simulink model "PMSM_MaxEfficiency"  (R2015a)
settings: Solver=ode45  StartTime=0.0  StopTime=5  RelTol=1e-3
values from neighbouring files (symbols this model uses):
  Ld = 0.00019    [aaa.mat]    (also in param.m = 2e-05)
  Lq = 0.00051    [aaa.mat]    (also in param.m = 4e-05)
  Pn = 4    [param.m]
  R = 2e-3    (= 0.002)    [param.m]
undefined symbols (not defined in the file or in its folder): D, Ia_vec, J, Phia, torque_vec
settings Model: Creator=hamada  LastModifiedBy=hamada

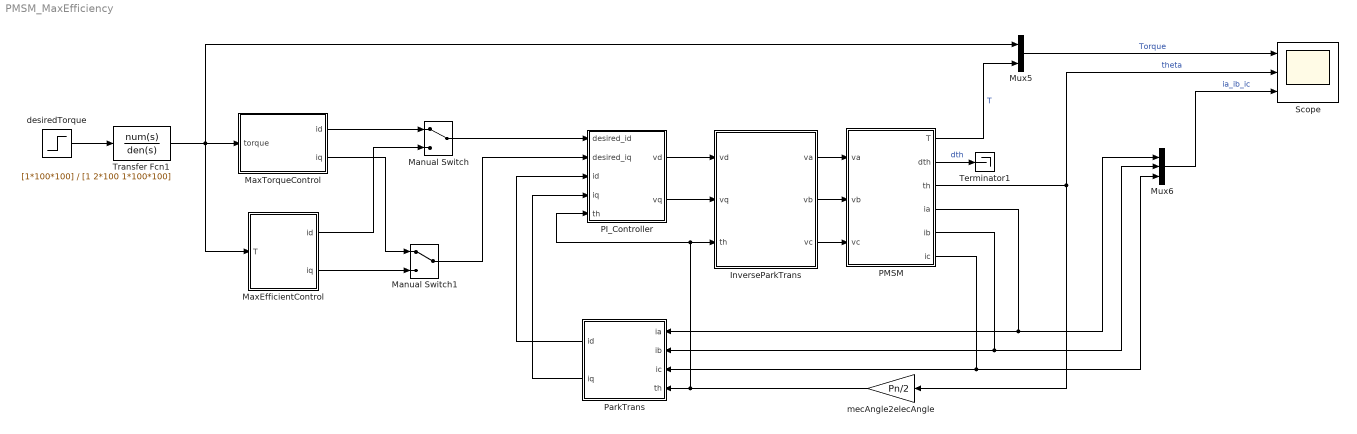
== system PMSM_MaxEfficiency ==
  InverseParkTrans : MATLAB Function  TreatAsAtomicUnit=on  SystemSampleTime=0.001
  Manual Switch : ManualSwitch
  Manual Switch1 : ManualSwitch
  MaxEfficientControl : MATLAB Function  TreatAsAtomicUnit=on  SystemSampleTime=0.001
  MaxTorqueControl : Subsystem
  Mux5 : Mux  Inputs=2
  Mux6 : Mux  Inputs=3
  PI_Controller : Subsystem  SystemSampleTime=0.001
  PMSM : Subsystem
  ParkTrans : MATLAB Function  TreatAsAtomicUnit=on
  Scope : Scope  NumInputPorts=3
      settings: TimeRange=5  YMin=0~0~-80  YMax=5~15~80
  Terminator1 : Terminator
  Transfer Fcn1 : TransferFcn  Numerator=[1*100*100]  Denominator=[1 2*100 1*100*100]
  desiredTorque : Step  After=5  SampleTime=0
  mecAngle2elecAngle : Gain  Gain=Pn/2
  wires:
  desiredTorque/1 -> Transfer Fcn1/1
  PMSM/1(T) -> Mux5/2  "T"
  PMSM/3(th) -> mecAngle2elecAngle/1, Scope/2  "theta"
  PMSM/4(ia) -> Mux6/1, ParkTrans/1(ia)
  PMSM/5(ib) -> ParkTrans/2(ib), Mux6/2
  PMSM/6(ic) -> ParkTrans/3(ic), Mux6/3
  InverseParkTrans/2(vb) -> PMSM/2(vb)
  InverseParkTrans/3(vc) -> PMSM/3(vc)
  InverseParkTrans/1(va) -> PMSM/1(va)
  mecAngle2elecAngle/1 -> ParkTrans/4(th), PI_Controller/5(th), InverseParkTrans/3(th)
  ParkTrans/1(id) -> PI_Controller/3(id)
  ParkTrans/2(iq) -> PI_Controller/4(iq)
  PI_Controller/1(vd) -> InverseParkTrans/1(vd)
  PI_Controller/2(vq) -> InverseParkTrans/2(vq)
  PMSM/2(dth) -> Terminator1/1  "dth"
  Mux5/1 -> Scope/1  "Torque"
  Mux6/1 -> Scope/3  "ia_ib_ic"
  Transfer Fcn1/1 -> MaxEfficientControl/1(T), MaxTorqueControl/1(torque), Mux5/1
  Manual Switch/1 -> PI_Controller/1(desired_id)
  MaxEfficientControl/2(iq) -> Manual Switch1/2
  MaxEfficientControl/1(id) -> Manual Switch/2
  MaxTorqueControl/1(id) -> Manual Switch/1
  MaxTorqueControl/2(iq) -> Manual Switch1/1
  Manual Switch1/1 -> PI_Controller/2(desired_iq)

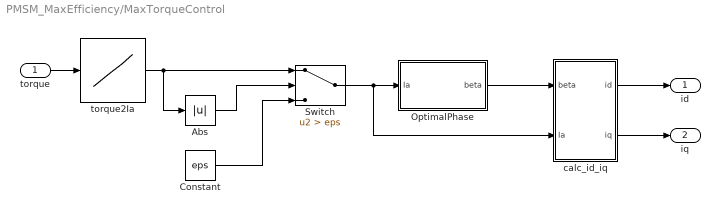
== system PMSM_MaxEfficiency/MaxTorqueControl ==
  torque : Inport
  Abs : Abs
  Constant : Constant  Value=eps
  OptimalPhase : Subsystem
  Switch : Switch  Criteria=u2 > Threshold  Threshold=eps
  calc_id_iq : Subsystem
  torque2Ia : Lookup_n-D  NumberOfTableDimensions=1  BreakpointsForDimension1=torque_vec  Table=Ia_vec  InternalRulePriority=Speed  RndMeth=Simplest  InputSameDT=on
  id : Outport
  iq : Outport  Port=2
  wires:
  torque/1 -> torque2Ia/1
  OptimalPhase/1(beta) -> calc_id_iq/1(beta)
  calc_id_iq/1(id) -> id/1
  calc_id_iq/2(iq) -> iq/1
  torque2Ia/1 -> Switch/1, Abs/1
  Abs/1 -> Switch/2
  Switch/1 -> calc_id_iq/2(Ia), OptimalPhase/1(Ia)
  Constant/1 -> Switch/3

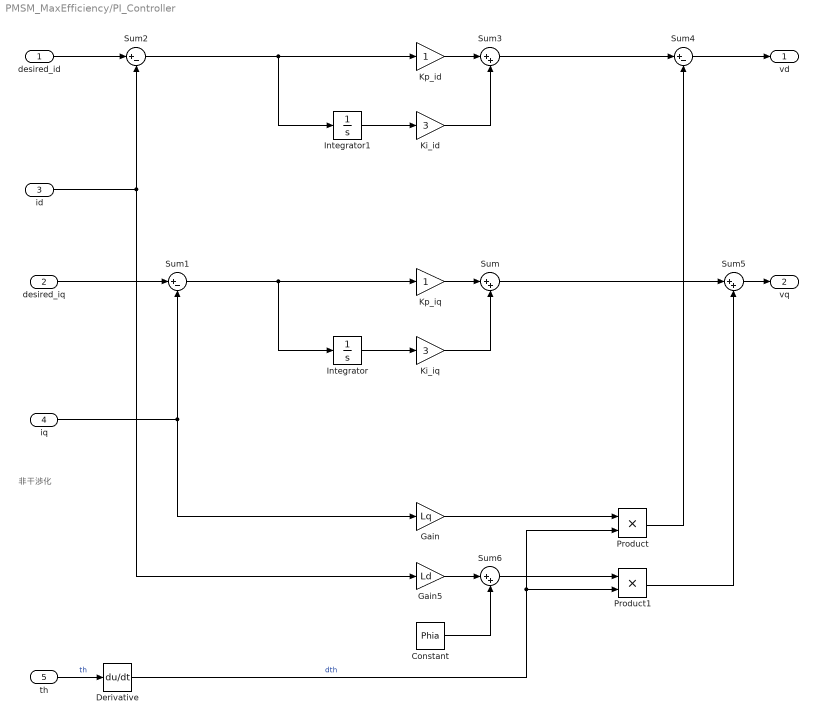
== system PMSM_MaxEfficiency/PI_Controller ==
  note: 非干渉化
  desired_id : Inport
  desired_iq : Inport  Port=2
  id : Inport  Port=3
  iq : Inport  Port=4
  th : Inport  Port=5
  Constant : Constant  Value=Phia
  Derivative : Derivative
  Gain : Gain  Gain=Lq
  Gain5 : Gain  Gain=Ld
  Integrator : Integrator
  Integrator1 : Integrator
  Ki_id : Gain  Gain=3
  Ki_iq : Gain  Gain=3
  Kp_id : Gain
  Kp_iq : Gain
  Product : Product
  Product1 : Product
  Sum{,3,5..6} (4 alike) : Sum  Inputs=|++
  Sum1 : Sum  Inputs=|+-
  Sum2 : Sum  Inputs=|+-
  Sum4 : Sum  Inputs=|+-
  vd : Outport
  vq : Outport  Port=2
  wires:
  Sum1/1 -> Integrator/1, Kp_iq/1
  desired_id/1 -> Sum2/1
  Kp_iq/1 -> Sum/1
  desired_iq/1 -> Sum1/1
  id/1 -> Sum2/2, Gain5/1
  iq/1 -> Sum1/2, Gain/1
  Sum/1 -> Sum5/1
  Integrator/1 -> Ki_iq/1
  Ki_iq/1 -> Sum/2
  Sum2/1 -> Integrator1/1, Kp_id/1
  Kp_id/1 -> Sum3/1
  Sum3/1 -> Sum4/1
  Integrator1/1 -> Ki_id/1
  Ki_id/1 -> Sum3/2
  th/1 -> Derivative/1  "th"
  Derivative/1 -> Product/2, Product1/2  "dth"
  Gain/1 -> Product/1
  Product/1 -> Sum4/2
  Sum4/1 -> vd/1
  Sum5/1 -> vq/1
  Gain5/1 -> Sum6/1
  Constant/1 -> Sum6/2
  Sum6/1 -> Product1/1
  Product1/1 -> Sum5/2

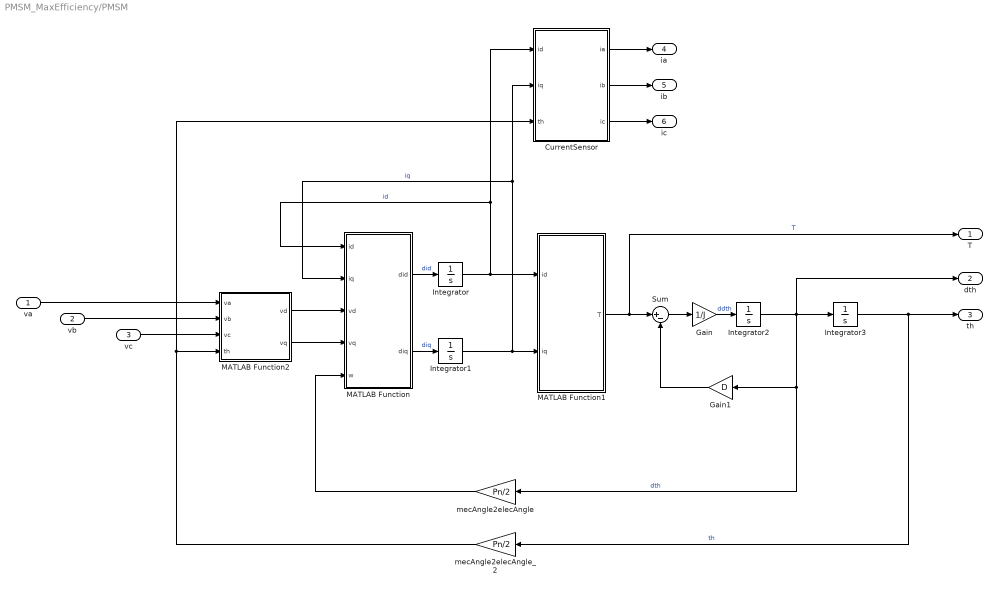
== system PMSM_MaxEfficiency/PMSM ==
  va : Inport
  vb : Inport  Port=2
  vc : Inport  Port=3
  CurrentSensor : MATLAB Function  TreatAsAtomicUnit=on
  Gain : Gain  Gain=1/J
  Gain1 : Gain  Gain=D
  Integrator{,1..3} (4 alike) : Integrator
  MATLAB Function : MATLAB Function  TreatAsAtomicUnit=on
  MATLAB Function1 : MATLAB Function  TreatAsAtomicUnit=on
  MATLAB Function2 : MATLAB Function  TreatAsAtomicUnit=on
  Sum : Sum  Inputs=|+-
  mecAngle2elecAngle : Gain  Gain=Pn/2
  mecAngle2elecAngle_2 : Gain  Gain=Pn/2
  T : Outport
  dth : Outport  Port=2
  th : Outport  Port=3
  ia : Outport  Port=4
  ib : Outport  Port=5
  ic : Outport  Port=6
  wires:
  CurrentSensor/3(ic) -> ic/1
  CurrentSensor/2(ib) -> ib/1
  CurrentSensor/1(ia) -> ia/1
  mecAngle2elecAngle_2/1 -> MATLAB Function2/4(th), CurrentSensor/3(th)
  mecAngle2elecAngle/1 -> MATLAB Function/5(w)
  Integrator3/1 -> mecAngle2elecAngle_2/1, th/1  "th"
  MATLAB Function2/2(vq) -> MATLAB Function/4(vq)
  MATLAB Function2/1(vd) -> MATLAB Function/3(vd)
  Gain1/1 -> Sum/2
  Integrator2/1 -> Gain1/1, mecAngle2elecAngle/1, Integrator3/1, dth/1  "dth"
  MATLAB Function1/1(T) -> Sum/1, T/1  "T"
  Gain/1 -> Integrator2/1  "ddth"
  Sum/1 -> Gain/1
  Integrator1/1 -> MATLAB Function1/2(iq), MATLAB Function/2(iq), CurrentSensor/2(iq)  "iq"
  Integrator/1 -> MATLAB Function1/1(id), MATLAB Function/1(id), CurrentSensor/1(id)  "id"
  MATLAB Function/2(diq) -> Integrator1/1  "diq"
  MATLAB Function/1(did) -> Integrator/1  "did"
  vc/1 -> MATLAB Function2/3(vc)
  vb/1 -> MATLAB Function2/2(vb)
  va/1 -> MATLAB Function2/1(va)

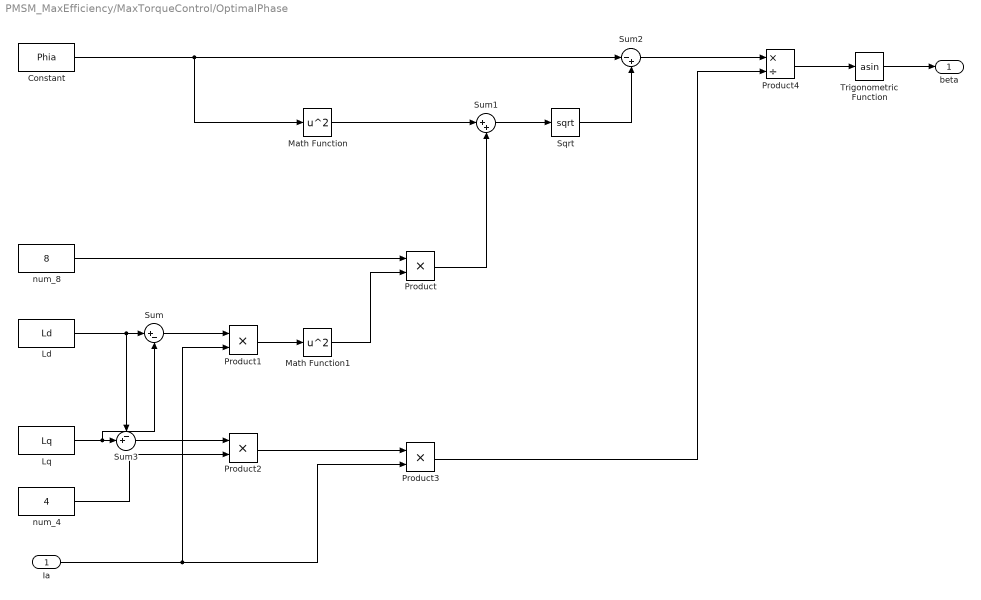
== system PMSM_MaxEfficiency/MaxTorqueControl/OptimalPhase ==
  Ia : Inport
  Constant : Constant  Value=Phia
  Ld : Constant  Value=Ld
  Lq : Constant  Value=Lq
  Math Function : Math  Operator=square  SaturateOnIntegerOverflow=on
  Math Function1 : Math  Operator=square  SaturateOnIntegerOverflow=on
  Product{,1..3} (4 alike) : Product
  Product4 : Product  Inputs=*/
  Sqrt : Sqrt  SaturateOnIntegerOverflow=on
  Sum : Sum  Inputs=|+-
  Sum1 : Sum  Inputs=|++
  Sum2 : Sum  Inputs=|-+
  Sum3 : Sum  Inputs=-+|
  Trigonometric Function : Trigonometry  Operator=asin
  num_4 : Constant  Value=4
  num_8 : Constant  Value=8
  beta : Outport
  wires:
  Constant/1 -> Sum2/1, Math Function/1
  Ld/1 -> Sum/1, Sum3/1
  Lq/1 -> Sum/2, Sum3/2
  Sum/1 -> Product1/1
  num_8/1 -> Product/1
  Math Function1/1 -> Product/2
  Product1/1 -> Math Function1/1
  Math Function/1 -> Sum1/1
  Product/1 -> Sum1/2
  Sum1/1 -> Sqrt/1
  Sqrt/1 -> Sum2/2
  Sum2/1 -> Product4/1
  Sum3/1 -> Product2/1
  Product2/1 -> Product3/1
  Ia/1 -> Product1/2, Product3/2
  num_4/1 -> Product2/2
  Product3/1 -> Product4/2
  Product4/1 -> Trigonometric Function/1
  Trigonometric Function/1 -> beta/1

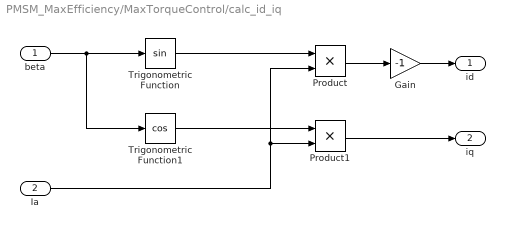
== system PMSM_MaxEfficiency/MaxTorqueControl/calc_id_iq ==
  beta : Inport
  Ia : Inport  Port=2
  Gain : Gain  Gain=-1
  Product : Product
  Product1 : Product
  Trigonometric Function : Trigonometry
  Trigonometric Function1 : Trigonometry  Operator=cos
  id : Outport
  iq : Outport  Port=2
  wires:
  Product/1 -> Gain/1
  beta/1 -> Trigonometric Function1/1, Trigonometric Function/1
  Trigonometric Function/1 -> Product/1
  Ia/1 -> Product1/2, Product/2
  Trigonometric Function1/1 -> Product1/1
  Product1/1 -> iq/1
  Gain/1 -> id/1

== matlab function PMSM_MaxEfficiency/InverseParkTrans ==
  data: vd input; vq input; va output; vb output; vc output; th input
function [ va, vb, vc ] = fcn( vd, vq, th ) 
    %#codegen
    buff = [
        cos( th ), -sin( th ), ( 1 / sqrt( 2 ) );
        cos( th - ( ( 2 * pi ) / 3 ) ), -sin( th - ( ( 2 * pi ) / 3 ) ), ( 1 / sqrt( 2 ) );
        cos( th + ( ( 2 * pi ) / 3 ) ), -sin( th + ( ( 2 * pi ) / 3 ) ), ( 1 / sqrt( 2 ) );
    ];

    vabc = sqrt( 2 / 3 ) * buff * [ vd;vq;0; ];
    va = vabc(1);
    vb = vabc(2);
    vc = vabc(3);
end

== matlab function PMSM_MaxEfficiency/ParkTrans ==
  data: ia input; ib input; ic input; th input; id output; iq output
function [ id, iq ] = fcn( ia, ib, ic, th ) 
    %#codegen
    buff = [
         cos( th ),  cos( th - ( ( 2 * pi ) / 3 ) ),  cos( th + ( ( 2 * pi ) / 3 ) );
        -sin( th ), -sin( th - ( ( 2 * pi ) / 3 ) ), -sin( th + ( ( 2 * pi ) / 3 ) );
        ( 1 / sqrt( 2 ) ), ( 1 / sqrt( 2 ) ), ( 1 / sqrt( 2 ) );
    ];

    idq = sqrt( 2 / 3 ) * buff * [ ia;ib;ic; ];
    id = idq(1);
    iq = idq(2);
end

== matlab function PMSM_MaxEfficiency/PMSM/MATLAB Function ==
  data: did output; diq output; id input; iq input; vd input; vq input; w input; R parameter; Ld parameter; Lq parameter; Phia parameter
function [ did, diq ] = fcn( id, iq, vd ,vq, w, R, Ld, Lq, Phia ) 
    %#codegen
    
    idq = [ id;iq; ];
    vdq = [ vd;vq; ];
    
    A = [ 
        -( R / Ld ), ( w * ( Lq / Ld ) );
        -( w * ( Ld / Lq ) ), -( R / Lq );
    ];
    
    B = [
        ( 1 / Ld ), 0;
        0, ( 1 / Lq );
    ];

    U = [
        0;
        -( w * ( Phia / Lq ) );
    ];

    didq = A * idq + B * vdq + U;
    
    did = didq(1);
    diq = didq(2);
end

== matlab function PMSM_MaxEfficiency/PMSM/MATLAB Function1 ==
  data: T output; id input; iq input; Ld parameter; Lq parameter; Phia parameter; Pn parameter
function T = fcn( id, iq, Ld, Lq, Phia, Pn ) 
    %#codegen
    
    T = ( Pn / 2 ) * ( Phia * iq + ( Ld - Lq ) * id * iq );

end

== matlab function PMSM_MaxEfficiency/PMSM/MATLAB Function2 ==
  data: va input; vb input; vc input; th input; vd output; vq output
function [ vd, vq ] = fcn( va, vb, vc, th ) 
    %#codegen
    buff = [
         cos( th ),  cos( th - ( ( 2 * pi ) / 3 ) ),  cos( th + ( ( 2 * pi ) / 3 ) );
        -sin( th ), -sin( th - ( ( 2 * pi ) / 3 ) ), -sin( th + ( ( 2 * pi ) / 3 ) );
        ( 1 / sqrt( 2 ) ), ( 1 / sqrt( 2 ) ), ( 1 / sqrt( 2 ) );
    ];

    vdq = sqrt( 2 / 3 ) * buff * [ va;vb;vc; ];
    vd = vdq(1);
    vq = vdq(2);
end

== matlab function PMSM_MaxEfficiency/PMSM/CurrentSensor ==
  data: id input; iq input; ia output; ib output; ic output; th input
function [ ia, ib, ic ] = fcn( id, iq, th ) 
    %#codegen
    buff = [
        cos( th ), -sin( th ), ( 1 / sqrt( 2 ) );
        cos( th - ( ( 2 * pi ) / 3 ) ), -sin( th - ( ( 2 * pi ) / 3 ) ), ( 1 / sqrt( 2 ) );
        cos( th + ( ( 2 * pi ) / 3 ) ), -sin( th + ( ( 2 * pi ) / 3 ) ), ( 1 / sqrt( 2 ) );
    ];

    iabc = sqrt( 2 / 3 ) * buff * [ id;iq;0; ];
    ia = iabc(1);
    ib = iabc(2);
    ic = iabc(3);
end

== matlab function PMSM_MaxEfficiency/MaxEfficientControl ==
  data: id output; iq output; T input; Pn parameter; Ld parameter; Lq parameter; Phia parameter
% ある目標トルクが与えられた際に，最も電流が小さくなるid, iqを実時間最適化によって計算する．
function [ id, iq ] = fcn( T, Pn, Ld, Lq, Phia ) 
    %#codegen
    % id=0の値を初期値とする
    var = [ 0;( ( 2 * T ) / ( Pn * Phia ) );0; ];
    
    % 初期値が最適解に近いので，3回程度でも収束する．
    for cnt = 1:10
        var = var - HessianMatrix( T, var(1), var(2), var(3), Pn, Ld, Lq, Phia ) \ GradVector( T, var(1), var(2), var(3), Pn, Ld, Lq, Phia );
    end
    
    id = var(1);
    iq = var(2);
end
